simulink model "test"  (R2020a)
settings: Solver=VariableStepAuto  StartTime=0.0  StopTime=10.0  RelTol=1e-3
values from neighbouring files (symbols this model uses):
  Be = 5    [Teleop_parameters.m]    (also in base.mat = 0.5; base_no_attrito.mat = 0.5; ci_siamo.mat; force_control.mat = 0.5)
  Bh = 0.02    [Teleop_parameters.m]    (also in base.mat; base_no_attrito.mat; ci_siamo.mat; force_control.mat)
  Fc_h = 5    [Teleop_parameters.m]    (also in base.mat; base_no_attrito.mat; ci_siamo.mat; force_control.mat)
  Jh = 0.02    [Teleop_parameters.m]    (also in base.mat; base_no_attrito.mat; ci_siamo.mat; force_control.mat)
  k_m = 19.34    [Teleop_parameters.m]    (also in base.mat; base_no_attrito.mat; ci_siamo.mat; force_control.mat)
  k_s = 19.34    [Teleop_parameters.m]    (also in base.mat; base_no_attrito.mat; ci_siamo.mat; force_control.mat)
  Kc2v_m = 2    [Teleop_parameters.m]    (also in base.mat; base_no_attrito.mat; ci_siamo.mat; force_control.mat)
  Kc2v_s = 2    [Teleop_parameters.m]    (also in base.mat; base_no_attrito.mat; ci_siamo.mat; force_control.mat)
  Kd_h = 0.5    [Teleop_parameters.m]    (also in base.mat = 1; base_no_attrito.mat = 1; ci_siamo.mat = 10; force_control.mat = 1)
  Kd_m = 0.005    [Teleop_parameters.m]    (also in base.mat = 1; base_no_attrito.mat = 1; ci_siamo.mat; force_control.mat = 1)
  Kd_s = 0.5    [Teleop_parameters.m]    (also in base.mat = 1; base_no_attrito.mat = 1; ci_siamo.mat; force_control.mat = 1)
  Ke = 10    [Teleop_parameters.m]    (also in base.mat; base_no_attrito.mat; ci_siamo.mat; force_control.mat)
  Kp_h = 1.2    [Teleop_parameters.m]    (also in base.mat; base_no_attrito.mat; ci_siamo.mat = 10; force_control.mat)
  Kp_m = 0.01    [Teleop_parameters.m]    (also in base.mat = 1; base_no_attrito.mat = 1; ci_siamo.mat; force_control.mat = 1)
  Kp_s = 1    [Teleop_parameters.m]    (also in base.mat; base_no_attrito.mat; ci_siamo.mat; force_control.mat)
  Kt2c_m = 1.182    [Teleop_parameters.m]    (also in base.mat; base_no_attrito.mat; ci_siamo.mat; force_control.mat)
  Kt2c_s = 1.182    [Teleop_parameters.m]    (also in base.mat; base_no_attrito.mat; ci_siamo.mat; force_control.mat)
  lArm_m = 0.1    [Teleop_parameters.m]    (also in base.mat; base_no_attrito.mat; ci_siamo.mat; force_control.mat)
  lArm_s = 0.1    [Teleop_parameters.m]    (also in base.mat; base_no_attrito.mat; ci_siamo.mat; force_control.mat)
  maxCurrent_m = 4.5    [Teleop_parameters.m]    (also in base.mat; base_no_attrito.mat; ci_siamo.mat; force_control.mat)
  maxCurrent_s = 4.5    [Teleop_parameters.m]    (also in base.mat; base_no_attrito.mat; ci_siamo.mat; force_control.mat)
  qe = 1.2    [Teleop_parameters.m]    (also in base.mat = 5; base_no_attrito.mat = 5; ci_siamo.mat = 0.5; force_control.mat = 5)
  tau_m = 1.217    [Teleop_parameters.m]    (also in base.mat; base_no_attrito.mat; ci_siamo.mat; force_control.mat)
  tau_s = 1.217    [Teleop_parameters.m]    (also in base.mat; base_no_attrito.mat; ci_siamo.mat; force_control.mat)
settings Model: Creator=giovanni  LastModifiedBy=giovanni

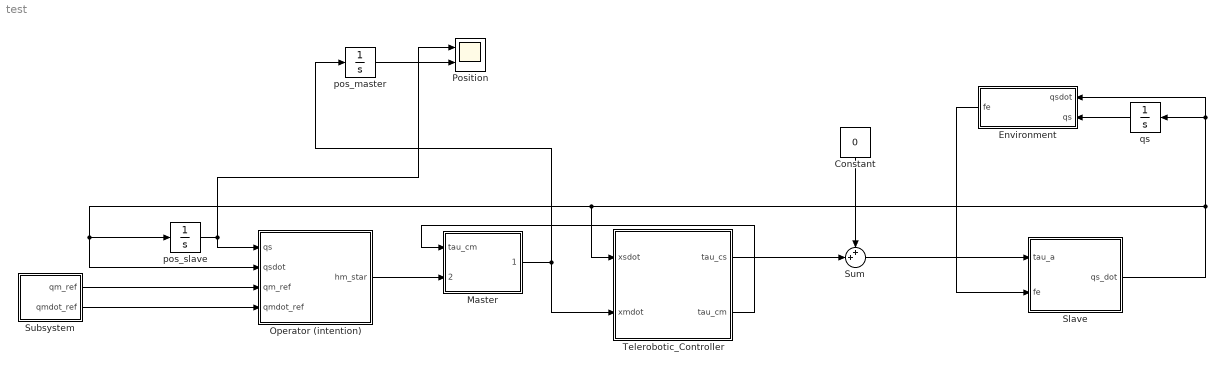
== system test ==
  Constant : Constant  Value=0
  Environment : Subsystem
  Master : Subsystem
  Operator (intention) : Subsystem
  Position : Scope  NumInputPorts=2
  Slave : Subsystem
  Subsystem : Subsystem
  Sum : Sum  Inputs=++|
  Telerobotic_Controller : Subsystem
  pos_master : Integrator
  pos_slave : Integrator
  qs : Integrator
  wires:
  Subsystem/1(qm_ref) -> Operator (intention)/3(qm_ref)
  Sum/1 -> Slave/1(tau_a)
  Telerobotic_Controller/1(tau_cs) -> Sum/2
  Telerobotic_Controller/2(tau_cm) -> Master/1(tau_cm)
  pos_master/1 -> Position/2
  Environment/1(fe) -> Slave/2(fe)
  Operator (intention)/1(hm_star) -> Master/2(hm_start)
  pos_slave/1 -> Operator (intention)/1(qs), Position/1
  Master/1(qm_dot) -> pos_master/1, Telerobotic_Controller/2(xmdot)
  qs/1 -> Environment/2(qs)
  Constant/1 -> Sum/1
  Subsystem/2(qmdot_ref) -> Operator (intention)/4(qmdot_ref)
  Slave/1(qs_dot) -> qs/1, Environment/1(qsdot), Telerobotic_Controller/1(xsdot), pos_slave/1, Operator (intention)/2(qsdot)

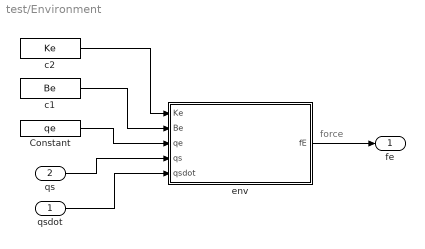
== system test/Environment ==
  note: force
  qsdot : Inport
  qs : Inport  Port=2
  Constant : Constant  Value=qe  SampleTime=0
  c1 : Constant  Value=Be  SampleTime=0
  c2 : Constant  Value=Ke  SampleTime=0
  env : MATLAB Function  TreatAsAtomicUnit=on
  fe : Outport  VectorParamsAs1DForOutWhenUnconnected=off
  wires:
  Constant/1 -> env/3(qe)
  c1/1 -> env/2(Be)
  c2/1 -> env/1(Ke)
  qs/1 -> env/4(qs)
  qsdot/1 -> env/5(qsdot)
  env/1(fE) -> fe/1

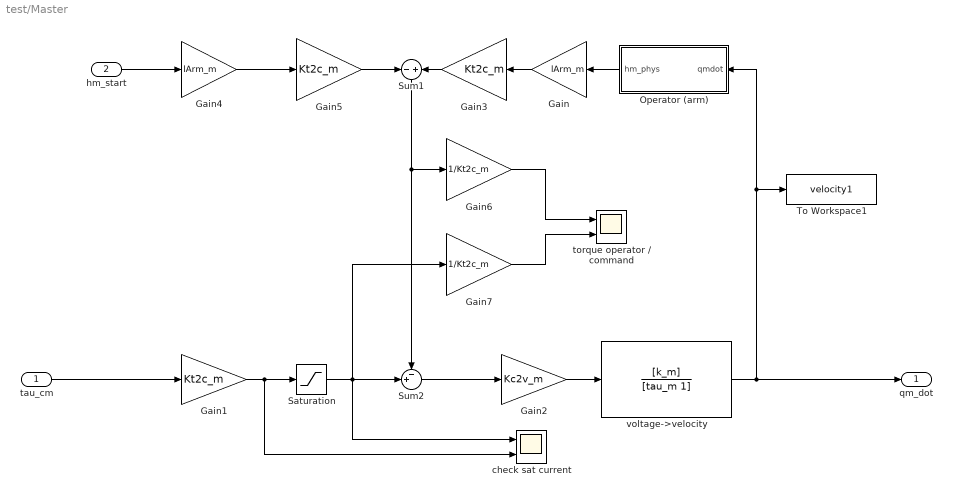
== system test/Master ==
  tau_cm : Inport
  hm_start : Inport  Port=2
  Gain : Gain  Gain=lArm_m
  Gain1 : Gain  Gain=Kt2c_m
  Gain2 : Gain  Gain=Kc2v_m
  Gain3 : Gain  Gain=Kt2c_m
  Gain4 : Gain  Gain=lArm_m
  Gain5 : Gain  Gain=Kt2c_m
  Gain6 : Gain  Gain=1/Kt2c_m
  Gain7 : Gain  Gain=1/Kt2c_m
  Operator (arm) : Subsystem
  Saturation : Saturate  UpperLimit=maxCurrent_m  LowerLimit=-maxCurrent_m
  Sum1 : Sum  Inputs=-+
  Sum2 : Sum  Inputs=-+|
  To Workspace1 : ToWorkspace  VariableName=velocity1  SaveFormat=Timeseries  SampleTime=-1
  check sat current : Scope  NumInputPorts=2
  torque operator / command : Scope  NumInputPorts=2
  voltage->velocity : TransferFcn  Numerator=[k_m]  Denominator=[tau_m 1]
  qm_dot : Outport
  wires:
  Gain7/1 -> torque operator / command/2
  Gain3/1 -> Sum1/2
  Operator (arm)/1(hm_phys) -> Gain/1
  voltage->velocity/1 -> qm_dot/1, Operator (arm)/1(qmdot), To Workspace1/1
  Gain4/1 -> Gain5/1
  Gain2/1 -> voltage->velocity/1
  Gain/1 -> Gain3/1
  Gain6/1 -> torque operator / command/1
  Gain5/1 -> Sum1/1
  Saturation/1 -> Gain7/1, Sum2/2, check sat current/1
  Sum1/1 -> Sum2/1, Gain6/1
  Sum2/1 -> Gain2/1
  Gain1/1 -> check sat current/2, Saturation/1
  tau_cm/1 -> Gain1/1
  hm_start/1 -> Gain4/1

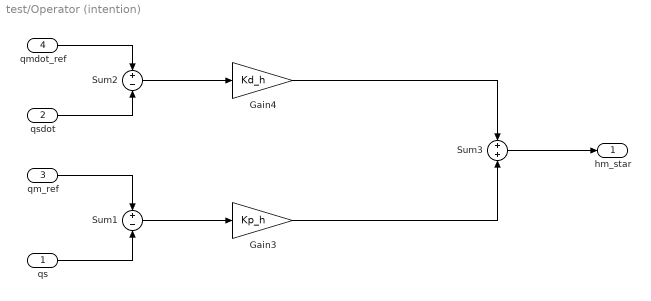
== system test/Operator (intention) ==
  qs : Inport
  qsdot : Inport  Port=2
  qm_ref : Inport  Port=3
  qmdot_ref : Inport  Port=4
  Gain3 : Gain  Gain=Kp_h
  Gain4 : Gain  Gain=Kd_h
  Sum1 : Sum  Inputs=+|-
  Sum2 : Sum  Inputs=+|-
  Sum3 : Sum  Inputs=+|+
  hm_star : Outport  VectorParamsAs1DForOutWhenUnconnected=off
  wires:
  qs/1 -> Sum1/2
  qm_ref/1 -> Sum1/1
  qmdot_ref/1 -> Sum2/1
  Sum1/1 -> Gain3/1
  qsdot/1 -> Sum2/2
  Sum2/1 -> Gain4/1
  Gain4/1 -> Sum3/1
  Gain3/1 -> Sum3/2
  Sum3/1 -> hm_star/1

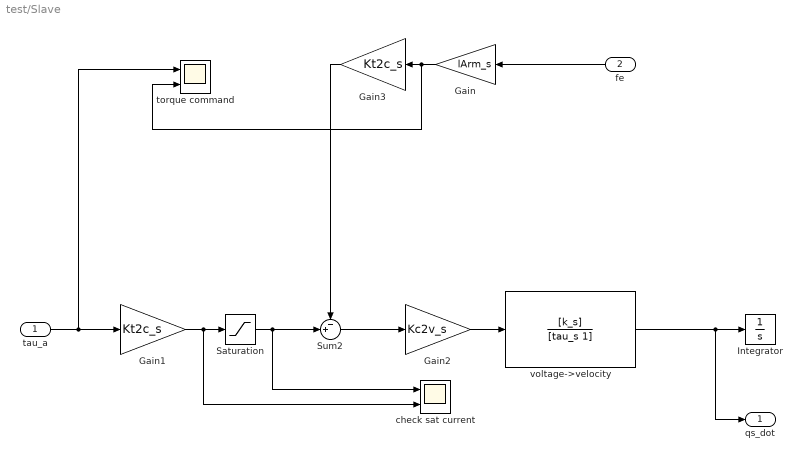
== system test/Slave ==
  tau_a : Inport
  fe : Inport  Port=2
  Gain : Gain  Gain=lArm_s
  Gain1 : Gain  Gain=Kt2c_s
  Gain2 : Gain  Gain=Kc2v_s
  Gain3 : Gain  Gain=Kt2c_s
  Integrator : Integrator
  Saturation : Saturate  UpperLimit=maxCurrent_s  LowerLimit=-maxCurrent_s
  Sum2 : Sum  Inputs=-+|
  check sat current : Scope  NumInputPorts=2
  torque command : Scope  NumInputPorts=2
  voltage->velocity : TransferFcn  Numerator=[k_s]  Denominator=[tau_s 1]
  qs_dot : Outport
  wires:
  Gain2/1 -> voltage->velocity/1
  Gain/1 -> torque command/2, Gain3/1
  Gain1/1 -> check sat current/2, Saturation/1
  Saturation/1 -> Sum2/2, check sat current/1
  Sum2/1 -> Gain2/1
  Gain3/1 -> Sum2/1
  voltage->velocity/1 -> qs_dot/1, Integrator/1
  tau_a/1 -> torque command/1, Gain1/1
  fe/1 -> Gain/1

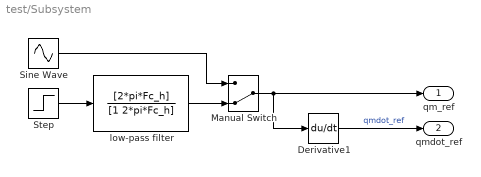
== system test/Subsystem ==
  Derivative1 : Derivative  CoefficientInTFapproximation=0.001
  Manual Switch : ManualSwitch  CurrentSetting=0
  Sine Wave : Sin  SampleTime=0
  Step : Step  SampleTime=0
  low-pass filter : TransferFcn  Numerator=[2*pi*Fc_h]  Denominator=[1 2*pi*Fc_h]
  qm_ref : Outport
  qmdot_ref : Outport  Port=2
  wires:
  low-pass filter/1 -> Manual Switch/2
  Manual Switch/1 -> qm_ref/1, Derivative1/1
  Derivative1/1 -> qmdot_ref/1  "qmdot_ref"
  Step/1 -> low-pass filter/1
  Sine Wave/1 -> Manual Switch/1

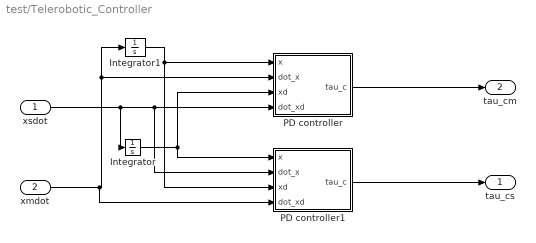
== system test/Telerobotic_Controller ==
  xsdot : Inport
  xmdot : Inport  Port=2
  Integrator : Integrator
  Integrator1 : Integrator
  PD controller : Subsystem
  PD controller1 : Subsystem
  tau_cs : Outport
  tau_cm : Outport  Port=2
  wires:
  Integrator/1 -> PD controller1/1(x), PD controller/3(xd)
  Integrator1/1 -> PD controller1/3(xd), PD controller/1(x)
  xsdot/1 -> PD controller1/2(dot_x), PD controller/4(dot_xd), Integrator/1
  xmdot/1 -> PD controller1/4(dot_xd), PD controller/2(dot_x), Integrator1/1
  PD controller/1(tau_c) -> tau_cm/1
  PD controller1/1(tau_c) -> tau_cs/1

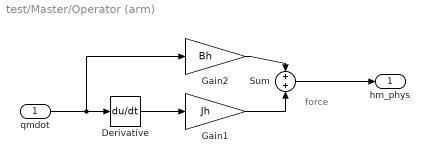
== system test/Master/Operator (arm) ==
  note: force
  qmdot : Inport
  Derivative : Derivative  CoefficientInTFapproximation=0.001
  Gain1 : Gain  Gain=Jh
  Gain2 : Gain  Gain=Bh
  Sum : Sum  Inputs=+|+
  hm_phys : Outport  VectorParamsAs1DForOutWhenUnconnected=off
  wires:
  qmdot/1 -> Gain2/1, Derivative/1
  Sum/1 -> hm_phys/1
  Derivative/1 -> Gain1/1
  Gain2/1 -> Sum/1
  Gain1/1 -> Sum/2

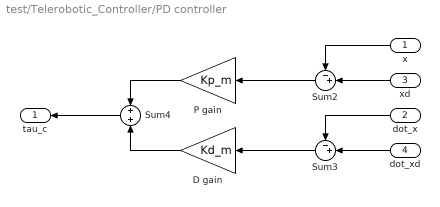
== system test/Telerobotic_Controller/PD controller ==
  x : Inport
  dot_x : Inport  Port=2
  xd : Inport  Port=3
  dot_xd : Inport  Port=4
  D gain : Gain  Gain=Kd_m
  P gain : Gain  Gain=Kp_m
  Sum2 : Sum  Inputs=-+|
  Sum3 : Sum  Inputs=-+|
  Sum4 : Sum
  tau_c : Outport  VectorParamsAs1DForOutWhenUnconnected=off
  wires:
  D gain/1 -> Sum4/2
  dot_x/1 -> Sum3/1
  dot_xd/1 -> Sum3/2
  x/1 -> Sum2/1
  xd/1 -> Sum2/2
  Sum3/1 -> D gain/1
  P gain/1 -> Sum4/1
  Sum4/1 -> tau_c/1
  Sum2/1 -> P gain/1

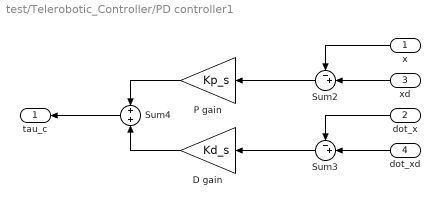
== system test/Telerobotic_Controller/PD controller1 ==
  x : Inport
  dot_x : Inport  Port=2
  xd : Inport  Port=3
  dot_xd : Inport  Port=4
  D gain : Gain  Gain=Kd_s
  P gain : Gain  Gain=Kp_s
  Sum2 : Sum  Inputs=-+|
  Sum3 : Sum  Inputs=-+|
  Sum4 : Sum
  tau_c : Outport  VectorParamsAs1DForOutWhenUnconnected=off
  wires:
  D gain/1 -> Sum4/2
  dot_x/1 -> Sum3/1
  dot_xd/1 -> Sum3/2
  x/1 -> Sum2/1
  xd/1 -> Sum2/2
  Sum3/1 -> D gain/1
  P gain/1 -> Sum4/1
  Sum4/1 -> tau_c/1
  Sum2/1 -> P gain/1

== matlab function test/Environment/env ==
  data: Ke input; Be input; qe input; qs input; fE output; qsdot input
function fE  = environment(Ke, Be, qe, qs, qsdot)
if qs > qe
   fE = Ke * (qs - qe) + Be * qsdot;
else
   fE = 0;
end
